simulink model "CSD_Segway_Nonlinear_with_Observer"  (R2018b)
settings: Solver=ode5  StartTime=0.0  StopTime=5  FixedStep=1e-4  RelTol=1e-3
values from neighbouring files (symbols this model uses):
  A = [0      1       0       0       0       0 ... (first row only)    [CSD_project.m]
  alpha = n * k_t / R_m    (= 0.0446559297218)    [CSD_project.m]
  B = [0     0 ... (first row only)    [CSD_project.m]
  beta = n * k_t * k_b /R_m + f_m    (= 0.0270286969253)    [CSD_project.m]
  C_obsv = eye(6)    [CSD_project.m]
  D_obsv = zeros(6, size(B,2)+size(C_obsv,1))    [CSD_project.m]
  f_w = 0    [CSD_project.m]
  g = 9.81    [CSD_project.m]
  J_m = 10^(-5)    (= 1e-05)    [CSD_project.m]
  K = place(A, B, 1e2*[-5,      -1, -0.8, -0.8,      -2e-2, -2e-2])    [CSD_project.m]
  L = 0.125    [CSD_project.m]
  L_obsv = L_obsv * alpha_obsv    [CSD_project.m]
  M = 0.6    [CSD_project.m]
  m_1 = (2 * m + M) * R^2 + 2 * J_w + 2 * n^2 * J_m    (= 0.00056096)    [CSD_project.m]
  m_3 = M * L^2 + J_psi + 2 * n^2 * J_m    (= 0.01252)    [CSD_project.m]
  m_4 = m * W^2 /2 + J_phi + W^2 / 2 / R^2 * (J_w + n^2 * J_m)    (= 0.00149726)    [CSD_project.m]
  n = 1    [CSD_project.m]
  observer_init = [0; 0; 0; 0; 0; 0]    [CSD_project.m]
  phi_init = pi/18    (= 0.174532925199)    [CSD_project.m]
  psi_init = pi/36    (= 0.0872664625997)    [CSD_project.m]
  R = 0.028    [CSD_project.m]
  theta_init = pi/18    (= 0.174532925199)    [CSD_project.m]
  W = 0.126    [CSD_project.m]
settings Model: Creator=sh  LastModifiedBy=shiha

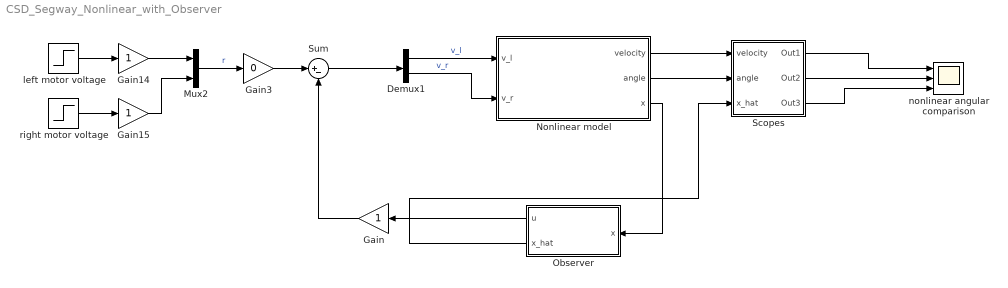
== system CSD_Segway_Nonlinear_with_Observer ==
  Demux1 : Demux  Outputs=2
  Gain : Gain
  Gain14 : Gain
  Gain15 : Gain
  Gain3 : Gain  Gain=0
  Mux2 : Mux  Inputs=2
  Nonlinear model : Subsystem
  Observer : Subsystem
  Scopes : Subsystem
  Sum : Sum  Inputs=|+-
  left motor voltage : Step  SampleTime=0
  nonlinear angular comparison : Scope  NumInputPorts=3
  right motor voltage : Step  SampleTime=0
  wires:
  left motor voltage/1 -> Gain14/1
  Mux2/1 -> Gain3/1  "r"
  Gain14/1 -> Mux2/1
  right motor voltage/1 -> Gain15/1
  Gain3/1 -> Sum/1
  Sum/1 -> Demux1/1
  Gain15/1 -> Mux2/2
  Demux1/1 -> Nonlinear model/1(v_l)  "v_l"
  Demux1/2 -> Nonlinear model/2(v_r)  "v_r"
  Nonlinear model/1(velocity) -> Scopes/1(velocity)
  Nonlinear model/2(angle) -> Scopes/2(angle)
  Scopes/2(Out2) -> nonlinear angular comparison/2
  Scopes/1(Out1) -> nonlinear angular comparison/1
  Scopes/3(Out3) -> nonlinear angular comparison/3
  Nonlinear model/3(x) -> Observer/1(x)
  Observer/1(u) -> Gain/1
  Observer/2(x_hat) -> Scopes/3(x_hat)
  Gain/1 -> Sum/2

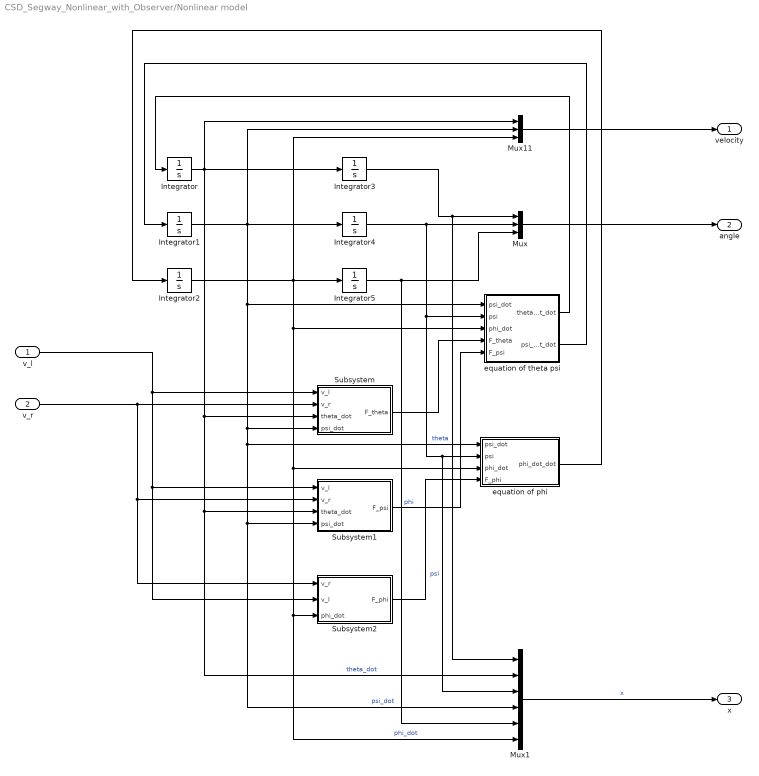
== system CSD_Segway_Nonlinear_with_Observer/Nonlinear model ==
  v_l : Inport
  v_r : Inport  Port=2
  Integrator : Integrator
  Integrator1 : Integrator
  Integrator2 : Integrator
  Integrator3 : Integrator  InitialCondition=theta_init
  Integrator4 : Integrator  InitialCondition=psi_init
  Integrator5 : Integrator  InitialCondition=phi_init
  Mux : Mux  Inputs=3
  Mux1 : Mux  Inputs=6
  Mux11 : Mux  Inputs=3
  Subsystem : Subsystem
  Subsystem1 : Subsystem
  Subsystem2 : Subsystem
  equation of phi : Subsystem
  equation of theta psi : Subsystem
  velocity : Outport
  angle : Outport  Port=2
  x : Outport  Port=3
  wires:
  Mux11/1 -> velocity/1
  Subsystem1/1(F_psi) -> equation of theta psi/5(F_psi)
  equation of phi/1(phi_dot_dot) -> Integrator2/1
  Mux/1 -> angle/1
  Integrator4/1 -> Mux1/3, equation of phi/2(psi), equation of theta psi/2(psi), Mux/2  "psi"
  Integrator2/1 -> Mux11/3, equation of theta psi/3(phi_dot), equation of phi/3(phi_dot), Mux1/6, Subsystem2/3(phi_dot), Integrator5/1  "phi_dot"
  Integrator3/1 -> Mux/1, Mux1/1  "theta"
  equation of theta psi/1(theta_dot_dot) -> Integrator/1
  Integrator/1 -> Mux11/1, Mux1/2, Subsystem1/3(theta_dot), Subsystem/3(theta_dot), Integrator3/1  "theta_dot"
  Subsystem/1(F_theta) -> equation of theta psi/4(F_theta)
  v_r/1 -> Subsystem2/1(v_r), Subsystem1/2(v_r), Subsystem/2(v_r)
  Integrator5/1 -> Mux/3, Mux1/5  "phi"
  equation of theta psi/2(psi_dot_dot) -> Integrator1/1
  Mux1/1 -> x/1  "x"
  v_l/1 -> Subsystem2/2(v_l), Subsystem1/1(v_l), Subsystem/1(v_l)
  Subsystem2/1(F_phi) -> equation of phi/4(F_phi)
  Integrator1/1 -> Mux11/2, equation of theta psi/1(psi_dot), equation of phi/1(psi_dot), Mux1/4, Subsystem1/4(psi_dot), Subsystem/4(psi_dot), Integrator4/1  "psi_dot"

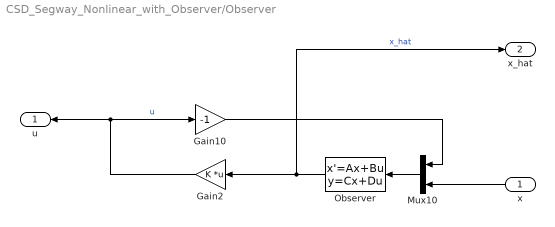
== system CSD_Segway_Nonlinear_with_Observer/Observer ==
  x : Inport
  Gain10 : Gain  Gain=-1
  Gain2 : Gain  Gain=K  Multiplication=Matrix(K*u)
  Mux10 : Mux  Inputs=2
  Observer : StateSpace  A=A - L_obsv * C_obsv  B=[B L_obsv]  C=eye(6)  D=D_obsv  InitialCondition=observer_init
  u : Outport
  x_hat : Outport  Port=2
  wires:
  Gain2/1 -> u/1, Gain10/1  "u"
  Mux10/1 -> Observer/1
  Gain10/1 -> Mux10/1
  x/1 -> Mux10/2
  Observer/1 -> x_hat/1, Gain2/1  "x_hat"

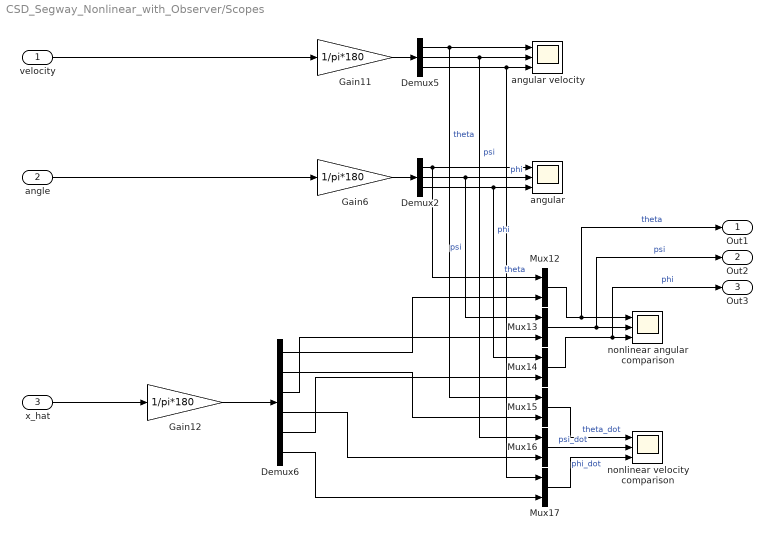
== system CSD_Segway_Nonlinear_with_Observer/Scopes ==
  velocity : Inport
  angle : Inport  Port=2
  x_hat : Inport  Port=3
  Demux2 : Demux  Outputs=3
  Demux5 : Demux  Outputs=3
  Demux6 : Demux  Outputs=6
  Gain11 : Gain  Gain=1/pi*180
  Gain12 : Gain  Gain=1/pi*180
  Gain6 : Gain  Gain=1/pi*180
  Mux{12..17} (6 alike) : Mux  Inputs=2
  angular : Scope  NumInputPorts=3
  angular velocity : Scope  NumInputPorts=3
  nonlinear angular comparison : Scope  NumInputPorts=3
  nonlinear velocity comparison : Scope  NumInputPorts=3
  Out1 : Outport
  Out2 : Outport  Port=2
  Out3 : Outport  Port=3
  wires:
  Demux2/1 -> angular/1, Mux12/1  "theta"
  angle/1 -> Gain6/1
  Demux6/5 -> Mux14/2
  Gain6/1 -> Demux2/1
  Mux17/1 -> nonlinear velocity comparison/3  "phi_dot"
  Gain12/1 -> Demux6/1
  Mux13/1 -> Out2/1, nonlinear angular comparison/2  "psi"
  Mux15/1 -> nonlinear velocity comparison/1  "theta_dot"
  Demux6/4 -> Mux16/2
  Demux6/3 -> Mux13/2
  Demux5/2 -> angular velocity/2, Mux16/1  "psi"
  Demux6/6 -> Mux17/2
  Demux2/2 -> angular/2, Mux13/1  "psi"
  Demux5/1 -> angular velocity/1, Mux15/1  "theta"
  Mux14/1 -> Out3/1, nonlinear angular comparison/3  "phi"
  Demux6/1 -> Mux12/2
  x_hat/1 -> Gain12/1
  Demux5/3 -> Mux17/1, angular velocity/3  "phi"
  Gain11/1 -> Demux5/1
  Mux12/1 -> Out1/1, nonlinear angular comparison/1  "theta"
  velocity/1 -> Gain11/1
  Demux6/2 -> Mux15/2
  Demux2/3 -> angular/3, Mux14/1  "phi"
  Mux16/1 -> nonlinear velocity comparison/2  "psi_dot"

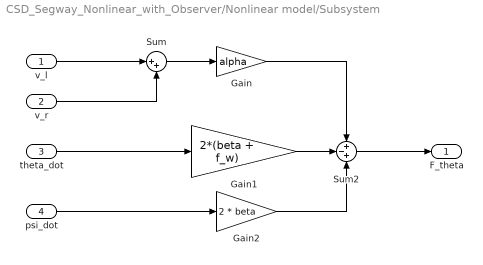
== system CSD_Segway_Nonlinear_with_Observer/Nonlinear model/Subsystem ==
  v_l : Inport
  v_r : Inport  Port=2
  theta_dot : Inport  Port=3
  psi_dot : Inport  Port=4
  Gain : Gain  Gain=alpha
  Gain1 : Gain  Gain=2*(beta + f_w)
  Gain2 : Gain  Gain=2 * beta
  Sum : Sum  Inputs=|++
  Sum2 : Sum  Inputs=+-+
  F_theta : Outport
  wires:
  v_l/1 -> Sum/1
  theta_dot/1 -> Gain1/1
  v_r/1 -> Sum/2
  Sum2/1 -> F_theta/1
  Gain1/1 -> Sum2/2
  Gain/1 -> Sum2/1
  Sum/1 -> Gain/1
  psi_dot/1 -> Gain2/1
  Gain2/1 -> Sum2/3

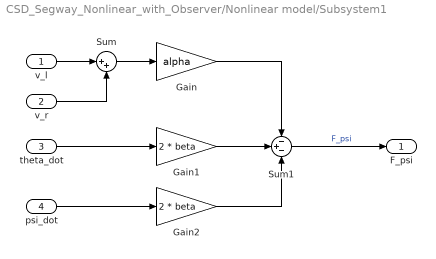
== system CSD_Segway_Nonlinear_with_Observer/Nonlinear model/Subsystem1 ==
  v_l : Inport
  v_r : Inport  Port=2
  theta_dot : Inport  Port=3
  psi_dot : Inport  Port=4
  Gain : Gain  Gain=alpha
  Gain1 : Gain  Gain=2 * beta
  Gain2 : Gain  Gain=2 * beta
  Sum : Sum  Inputs=|++
  Sum1 : Sum  Inputs=-+-
  F_psi : Outport
  wires:
  psi_dot/1 -> Gain2/1
  v_l/1 -> Sum/1
  Sum/1 -> Gain/1
  Sum1/1 -> F_psi/1  "F_psi"
  theta_dot/1 -> Gain1/1
  Gain/1 -> Sum1/1
  v_r/1 -> Sum/2
  Gain2/1 -> Sum1/3
  Gain1/1 -> Sum1/2

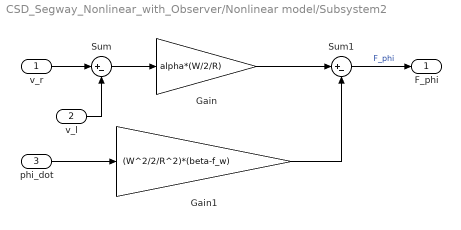
== system CSD_Segway_Nonlinear_with_Observer/Nonlinear model/Subsystem2 ==
  v_r : Inport
  v_l : Inport  Port=2
  phi_dot : Inport  Port=3
  Gain : Gain  Gain=alpha*(W/2/R)
  Gain1 : Gain  Gain=(W^2/2/R^2)*(beta-f_w)
  Sum : Sum  Inputs=|+-
  Sum1 : Sum  Inputs=|+-
  F_phi : Outport
  wires:
  Sum1/1 -> F_phi/1  "F_phi"
  phi_dot/1 -> Gain1/1
  v_l/1 -> Sum/2
  v_r/1 -> Sum/1
  Sum/1 -> Gain/1
  Gain/1 -> Sum1/1
  Gain1/1 -> Sum1/2

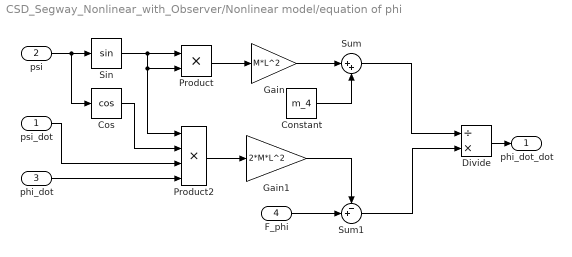
== system CSD_Segway_Nonlinear_with_Observer/Nonlinear model/equation of phi ==
  psi_dot : Inport
  psi : Inport  Port=2
  phi_dot : Inport  Port=3
  F_phi : Inport  Port=4
  Constant : Constant  Value=m_4
  Cos : Trigonometry  Operator=cos
  Divide : Product  Inputs=/*
  Gain : Gain  Gain=M*L^2
  Gain1 : Gain  Gain=2*M*L^2
  Product : Product
  Product2 : Product  Inputs=4
  Sin : Trigonometry
  Sum : Sum  Inputs=|++
  Sum1 : Sum  Inputs=-+|
  phi_dot_dot : Outport
  wires:
  psi_dot/1 -> Product2/3
  F_phi/1 -> Sum1/2
  Gain/1 -> Sum/1
  Constant/1 -> Sum/2
  Product2/1 -> Gain1/1
  Sum/1 -> Divide/1
  Gain1/1 -> Sum1/1
  psi/1 -> Cos/1, Sin/1
  Product/1 -> Gain/1
  Sum1/1 -> Divide/2
  phi_dot/1 -> Product2/4
  Cos/1 -> Product2/2
  Divide/1 -> phi_dot_dot/1
  Sin/1 -> Product/2, Product2/1, Product/1

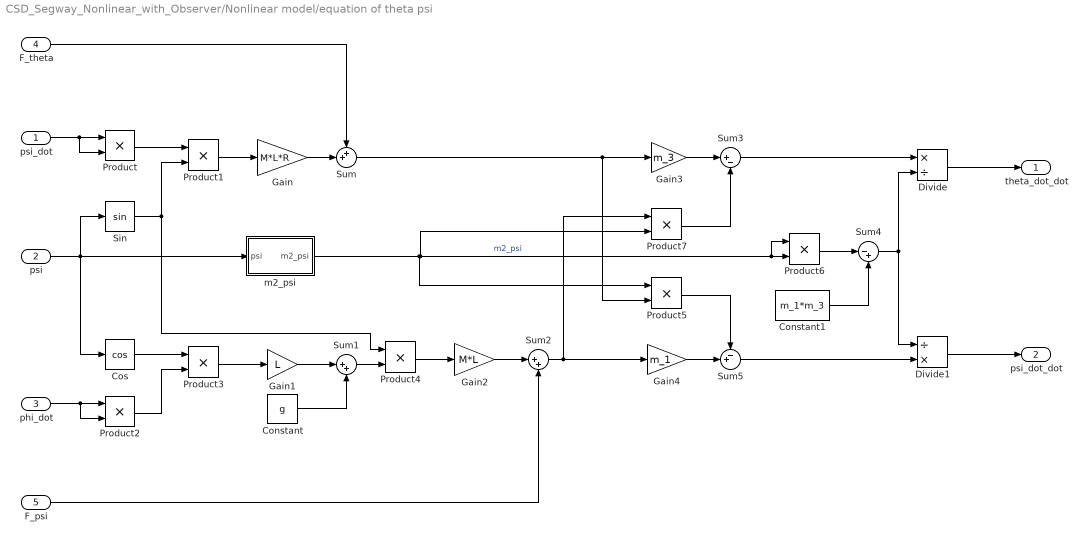
== system CSD_Segway_Nonlinear_with_Observer/Nonlinear model/equation of theta psi ==
  psi_dot : Inport
  psi : Inport  Port=2
  phi_dot : Inport  Port=3
  F_theta : Inport  Port=4
  F_psi : Inport  Port=5
  Constant : Constant  Value=g
  Constant1 : Constant  Value=m_1*m_3
  Cos : Trigonometry  Operator=cos
  Divide : Product  Inputs=*/
  Divide1 : Product  Inputs=/*
  Gain : Gain  Gain=M*L*R
  Gain1 : Gain  Gain=L
  Gain2 : Gain  Gain=M*L
  Gain3 : Gain  Gain=m_3
  Gain4 : Gain  Gain=m_1
  Product{,1..7} (8 alike) : Product
  Sin : Trigonometry
  Sum : Sum  Inputs=++|
  Sum1 : Sum  Inputs=|++
  Sum2 : Sum  Inputs=|++
  Sum3 : Sum  Inputs=|+-
  Sum4 : Sum  Inputs=|-+
  Sum5 : Sum  Inputs=-+|
  m2_psi : Subsystem
  theta_dot_dot : Outport
  psi_dot_dot : Outport  Port=2
  wires:
  Product2/1 -> Product3/2
  Product4/1 -> Gain2/1
  Gain2/1 -> Sum2/1
  Gain1/1 -> Sum1/1
  psi/1 -> Cos/1, m2_psi/1(psi), Sin/1
  F_psi/1 -> Sum2/2
  Product3/1 -> Gain1/1
  Sum1/1 -> Product4/2
  phi_dot/1 -> Product2/2, Product2/1
  Product1/1 -> Gain/1
  psi_dot/1 -> Product/2, Product/1
  Cos/1 -> Product3/1
  Product/1 -> Product1/1
  Constant/1 -> Sum1/2
  Sum/1 -> Product5/2, Gain3/1
  Sum2/1 -> Product7/1, Gain4/1
  Gain3/1 -> Sum3/1
  Product7/1 -> Sum3/2
  Sum3/1 -> Divide/1
  Product6/1 -> Sum4/1
  Constant1/1 -> Sum4/2
  m2_psi/1(m2_psi) -> Product6/1, Product6/2, Product7/2, Product5/1  "m2_psi"
  Gain4/1 -> Sum5/2
  Product5/1 -> Sum5/1
  Sum5/1 -> Divide1/2
  Sum4/1 -> Divide1/1, Divide/2
  Divide/1 -> theta_dot_dot/1
  Divide1/1 -> psi_dot_dot/1
  Gain/1 -> Sum/2
  F_theta/1 -> Sum/1
  Sin/1 -> Product1/2, Product4/1

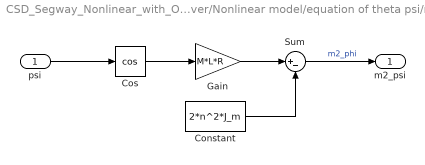
== system CSD_Segway_Nonlinear_with_Observer/Nonlinear model/equation of theta psi/m2_psi ==
  psi : Inport
  Constant : Constant  Value=2*n^2*J_m
  Cos : Trigonometry  Operator=cos
  Gain : Gain  Gain=M*L*R
  Sum : Sum  Inputs=|+-
  m2_psi : Outport
  wires:
  Gain/1 -> Sum/1
  psi/1 -> Cos/1
  Sum/1 -> m2_psi/1  "m2_phi"
  Cos/1 -> Gain/1
  Constant/1 -> Sum/2
